simulink model "tle2magField_util"  (R2018b)
settings: Solver=VariableStepAuto  StartTime=0.0  StopTime=6000  RelTol=1e-3
libraries: clock_lib x1, time_Lib x1, magField_lib x1, sgp4_lib_fsw x1
settings Model: Creator=taylorreynolds  LastModifiedBy=taylorreynolds

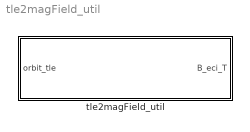
== system tle2magField_util ==
  tle2magField_util : Subsystem

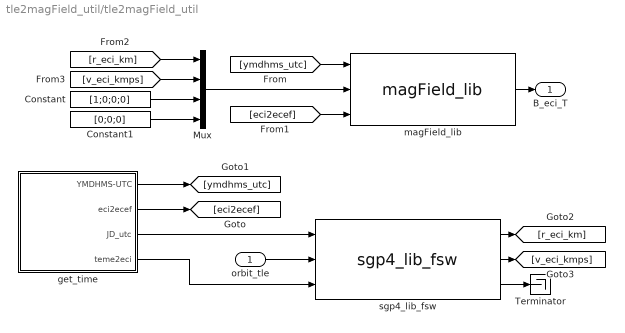
== system tle2magField_util/tle2magField_util ==
  orbit_tle : Inport
  Constant : Constant  Value=[1;0;0;0]
  Constant1 : Constant  Value=[0;0;0]
  Mux : Mux  Inputs=[3 3 4 3]
  Terminator : Terminator
  get_time : Subsystem
  magField_lib : magField_lib/magField_lib  SystemSampleTime=-1
  sgp4_lib_fsw : sgp4_lib_fsw/sgp4_lib_fsw  SystemSampleTime=-1
  B_eci_T : Outport
  wires:
  get_time/2(eci2ecef) -> [eci2ecef]
  Mux/1 -> magField_lib/2
  get_time/1(YMDHMS-UTC) -> [ymdhms_utc]
  magField_lib/1 -> B_eci_T/1
  sgp4_lib_fsw/3 -> Terminator/1
  get_time/3(JD_utc) -> sgp4_lib_fsw/1
  get_time/4(teme2eci) -> sgp4_lib_fsw/3
  orbit_tle/1 -> sgp4_lib_fsw/2
  [ymdhms_utc] -> magField_lib/1
  [eci2ecef] -> magField_lib/3
  sgp4_lib_fsw/1 -> [r_eci_km]
  sgp4_lib_fsw/2 -> [v_eci_kmps]
  [r_eci_km] -> Mux/1
  [v_eci_kmps] -> Mux/2
  Constant/1 -> Mux/3
  Constant1/1 -> Mux/4

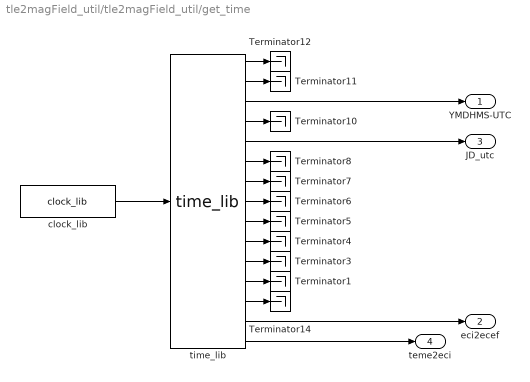
== system tle2magField_util/tle2magField_util/get_time ==
  Terminator{1,3..8,10..12,14} (11 alike) : Terminator
  clock_lib : clock_lib/clock_lib  SystemSampleTime=-1
  "time_lib " : time_Lib/time_lib    SystemSampleTime=-1
  YMDHMS-UTC : Outport
  eci2ecef : Outport  Port=2
  JD_utc : Outport  Port=3
  teme2eci : Outport  Port=4
  wires:
  clock_lib/1 -> "time_lib "/1
  "time_lib "/3 -> YMDHMS-UTC/1
  "time_lib "/14 -> eci2ecef/1
  "time_lib "/13 -> Terminator14/1
  "time_lib "/12 -> Terminator1/1
  "time_lib "/11 -> Terminator3/1
  "time_lib "/10 -> Terminator4/1
  "time_lib "/9 -> Terminator5/1
  "time_lib "/8 -> Terminator6/1
  "time_lib "/7 -> Terminator7/1
  "time_lib "/6 -> Terminator8/1
  "time_lib "/4 -> Terminator10/1
  "time_lib "/2 -> Terminator11/1
  "time_lib "/1 -> Terminator12/1
  "time_lib "/15 -> teme2eci/1
  "time_lib "/5 -> JD_utc/1
